simulink model "ECS787"  (R2013a)
settings: Solver=ode45  StartTime=0.0  StopTime=10000  RelTol=1e-3
InitFcn:
  | load('SampleOutput.mat')
  | 
  | load('SampleFuelBurn.mat')
undefined symbols (not defined in the file): AirProp
libraries: PowerFlowLib x8, simulink x4
(part 1 of 6)
settings Model: Creator=ASELab1  LastModifiedBy=ASELab1
settings DataIOCC: SignalLoggingSaveFormat=ModelDataLogs
settings DebuggingCC: MultiTaskDSMMsg=warning  MultiTaskCondExecSysMsg=none  StrictBusMsg=None
settings RTWCC: IncludeERTFirstTime=on

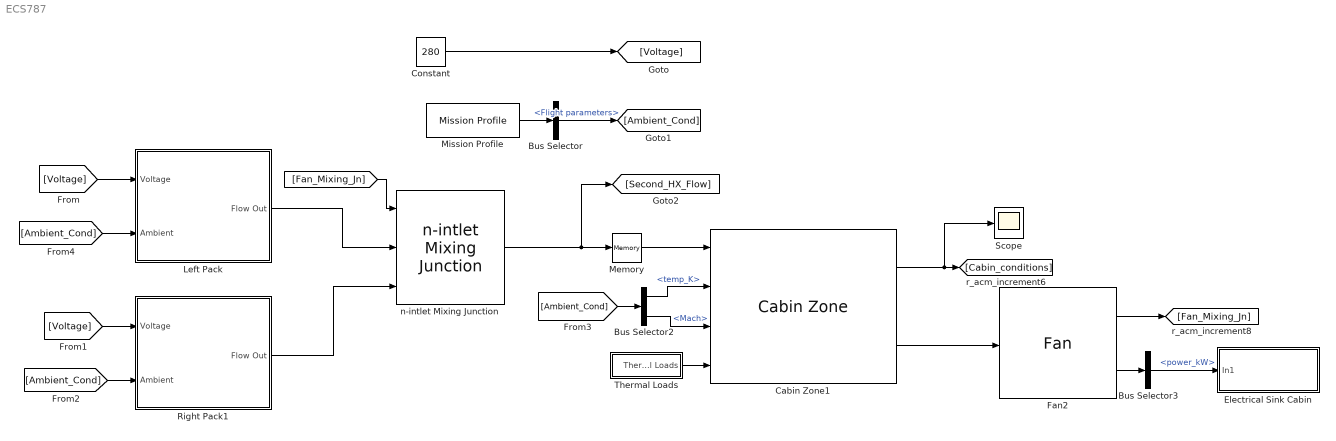
== system ECS787 ==
  Bus Selector : BusSelector  OutputSignals=Flight parameters
  Bus Selector2 : BusSelector  OutputSignals=temp_K,Mach
  Bus Selector3 : BusSelector  OutputSignals=power_kW
  Cabin Zone1 : PowerFlowLib/Energy & Power Systems/Thermal/ECS/Cabin Zone  A_fuselage=880  V_cab=245  n_pass=300  L_shell=0.003  K_shell=1  L_insulation=0.02  K_insulation=1  L_coating=0.002  K_coating=1  Vdot_sa_pass=0.009438  q_pass=60  RAR=.25  h_outside=1  h_inside=1
  Constant : Constant  Value=280
  Electrical Sink Cabin : Subsystem
  Fan2 : PowerFlowLib/Energy & Power Systems/Thermal/ECS/Fan  N_fan=1725
  Left Pack : Subsystem
  Memory : Memory
  Mission Profile : PowerFlowLib/Mission Profile/Mission Profile  mssn_check=off  mssn_prof=MSSN  del_P=0  del_T=0  del_rho=0  pres_msl=101.3  temp_msl=15  dens_msl=1.229
  Right Pack1 : Subsystem
  Scope : Scope
  Thermal Loads : Subsystem
  n-intlet Mixing Junction : PowerFlowLib/Energy & Power Systems/Thermal/ECS/n-intlet Mixing Junction  no_inlets=3  d_in_1=0.1  d_in_2=0.1  d_out=0.2
  wires:
  Mission Profile/1 -> Bus Selector/1
  Constant/1 -> [Voltage]
  Bus Selector/1 -> [Ambient_Cond]  "<Flight parameters>"
  Left Pack/1(Flow Out) -> n-intlet Mixing Junction/2
  Right Pack1/1(Flow Out) -> n-intlet Mixing Junction/3
  n-intlet Mixing Junction/1 -> [Second_HX_Flow], Memory/1
  Memory/1 -> Cabin Zone1/1
  [Ambient_Cond] -> Bus Selector2/1
  Bus Selector2/1 -> Cabin Zone1/2  "<temp_K>"
  Bus Selector2/2 -> Cabin Zone1/3  "<Mach>"
  Thermal Loads/1("Thermal Loads ") -> Cabin Zone1/4
  Cabin Zone1/2 -> Fan2/1
  Cabin Zone1/1 -> Scope/1, [Cabin_conditions]
  Fan2/2 -> Bus Selector3/1
  Bus Selector3/1 -> Electrical Sink Cabin/1(In1)  "<power_kW>"
  Fan2/1 -> [Fan_Mixing_Jn]
  [Fan_Mixing_Jn] -> n-intlet Mixing Junction/1
  [Voltage] -> Left Pack/1(Voltage)
  [Voltage] -> Right Pack1/1(Voltage)
  [Ambient_Cond] -> Left Pack/2(Ambient)
  [Ambient_Cond] -> Right Pack1/2(Ambient)

== system ECS787/Electrical Sink Cabin ==
  In1 : Inport

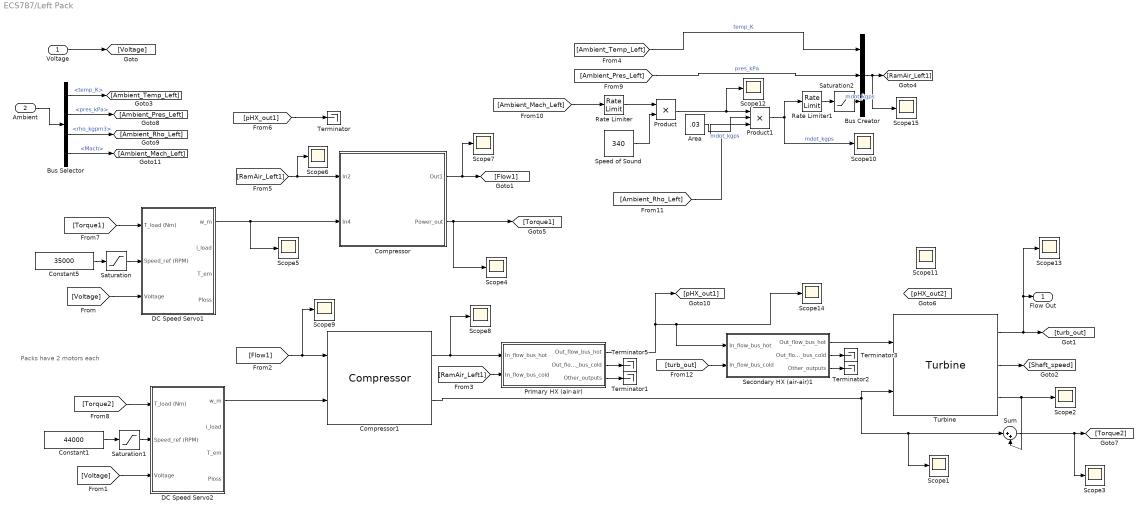
== system ECS787/Left Pack ==
  note: Packs have 2 motors each
  Voltage : Inport
  Ambient : Inport  Port=2
  "Area " : Constant  Value=.03
  Bus Creator : BusCreator  Inputs=3
  Bus Selector : BusSelector  OutputSignals=temp_K,pres_kPa,rho_kgpm3,Mach
  Compressor : Subsystem  AncestorBlock=PowerFlowLib/Energy & Power Systems/Thermal/ECS/Compressor
      mask help: COMPRESSOR (ECS)
      mask init:
      | load AirProp
      | load CompProp
      mask Help:
      | Main Assumptions
      | 1. The Turbine and the compressor are coupled to each other (turbocharger).
      | 2. Maps are provided to compute the efficiency of the compressor.
      | 3. There is no heat transfer from the compressor to the surrounding.
      mask Display:
      | image(imread('compressor.png'))
      | port_label('input',1,'{ \bfFlow In}','texmode','on')
      | port_label('input',2,'{ \bfShaft Speed}','texmode','on');
      | 
      | 
      | port_label('output',1,'{\bfFlow Out}','texmode','on')
      | port_label('output',2,'{\bfComp. Work}','texmode','on')
  Compressor1 : PowerFlowLib/Energy & Power Systems/Thermal/ECS/Compressor
      link override "m and P ": Gain=1
  Constant1 : Constant  Value=44000
  Constant5 : Constant  Value=35000
  DC Speed Servo1 : Subsystem  AncestorBlock=PowerFlowLib/Energy & Power Systems/Electrical/Machines/DC Speed Servo  mask{Vf=280, Ra=0.05, La=0.9e-3, Rfsh=400, Lfsh=320, Lmsh=1.9, J=1.5}
      mask prompts: Vf "Field voltage (V)"; Ra "Armature resistance (Ohms)"; La "Armature inductance (H)"; Rfsh "Shunt field resistance (Ohms)"; Lfsh "Shunt field inductance (H)"; Lmsh "Mutual inductance (H)"; J "Rotor moment of inertia (Kgm^2)"
  DC Speed Servo2 : Subsystem  AncestorBlock=PowerFlowLib/Energy & Power Systems/Electrical/Machines/DC Speed Servo  mask{Vf=280, Ra=0.05, La=0.9e-3, Rfsh=400, Lfsh=320, Lmsh=1.9, J=1.5}
      mask prompts: Vf "Field voltage (V)"; Ra "Armature resistance (Ohms)"; La "Armature inductance (H)"; Rfsh "Shunt field resistance (Ohms)"; Lfsh "Shunt field inductance (H)"; Lmsh "Mutual inductance (H)"; J "Rotor moment of inertia (Kgm^2)"
  Primary HX (air-air) : Subsystem  AncestorBlock=PowerFlowLib/Energy & Power Systems/Thermal/ECS/Air-Air HX  mask(Air-Air Heat Exchanger){L_hx=0.2, W_hx=0.2, H_hx=0.2, t_p=0.0008, K_p=167, cp_hx=883, m_cm=16, l_fin=.005, t_fin=0.0002, s_fin=0.0015, h_fin=0.0095, K_n=167, eta_f=0.8, T_cm_0=50}
      mask prompts: L_hx "Length of HX in the flow direction [m]"; W_hx "Width of HX [m]"; H_hx "Height of HX [m]"; t_p "HX plate thickness [m]"; K_p "Thermal conductivity of the plates [W/m.K]"; cp_hx "Specific heat of the HX material [J/kg.K]"; m_cm "Mass of HX [kg]"; l_fin "Fin length [m]"; t_fin "Fin thickness [m]"; s_fin "Fin free flow width [m]"; h_fin "Fin free flow height [m]"; K_n "Thermal conductivity of the fin material [W/m.K]"; eta_f "Fin efficiency"; T_cm_0 "Initial_HX_core_temp_[C]"
      mask init:
      | load AirProp
      mask Help:
      | Main Assumptions:
      | 
      | 1. Rectangular offset-strip fin heat exchanger.
      | 2. Lumped parameter model.
      | 3. Constant user-defined efficiency.
      | 4. Number of passages is the same for both the cold and hot fluid passages (usually
      | one of the flows has 1 more passage to reduce ambient losses).
      | 5. Similar plate and fin geometries for both the hot and cold fluid sides (the
      | objective is to simplify modeling and reduce the number of input parameters needed).
      | 6. Neglect heat transfer from fin face
      | 7. Neglect conduction heat transfer in the fin and plate bases
      mask Display:
      | port_label('input',1,'{ \bfFlow In (Hot)}','texmode','on')
      | port_label('input',2,'{ \bfFlow In (Cold)}','texmode','on');
      | 
      | port_label('output',1,'{\bfFlow Out (Hot)}','texmode','on')
      | port_label('output',2,'{\bfFlow Out (Cold)}','texmode','on')
      | port_label('output',3,'{\bfMisc. Data}','texmode','on')
  Product : Product
  Product1 : Product  Inputs=3
  Rate Limiter : RateLimiter  RisingSlewLimit=.02  FallingSlewLimit=-.02  SampleTimeMode=inherited
  Rate Limiter1 : RateLimiter  RisingSlewLimit=.02  FallingSlewLimit=-.02  SampleTimeMode=inherited
  Saturation : Saturate  UpperLimit=40000  LowerLimit=10000
  Saturation1 : Saturate  UpperLimit=60000  LowerLimit=30000
  Saturation2 : Saturate  UpperLimit=20  LowerLimit=.01
  Scope{1..15} (15 alike) : Scope
      Scope1 settings: YMin=469600  YMax=470800  SaveName=ScopeData6
      Scope10 settings: YMin=0  YMax=0.25  SaveName=ScopeData17
      Scope11 settings: YMin=-1750  YMax=500
      Scope12 settings: SaveName=ScopeData19
      Scope13 settings: YMin=0  YMax=750  SaveName=ScopeData2
      Scope14 settings: YMin=0  YMax=375  SaveName=ScopeData4
      Scope15 settings: YMin=0  YMax=300  SaveName=ScopeData5
      Scope2 settings: YMin=-2.5e+06  YMax=4e+06  SaveName=ScopeData7
      Scope3 settings: YMin=4.29e+06  YMax=4.3e+06  SaveName=ScopeData8
      Scope4 settings: SaveName=ScopeData9
      Scope5 settings: YMin=0  YMax=11000  SaveName=ScopeData10
      Scope6 settings: SaveName=ScopeData11
      Scope7 settings: TimeRange=10000  YMin=0  YMax=350  SaveName=ScopeData12
      Scope8 settings: YMin=0  YMax=850  SaveName=ScopeData13
      Scope9 settings: YMin=0  YMax=350  SaveName=ScopeData14
  Secondary HX (air-air)1 : Subsystem  AncestorBlock=PowerFlowLib/Energy & Power Systems/Thermal/ECS/Air-Air HX  mask(Air-Air Heat Exchanger){L_hx=0.2, W_hx=0.2, H_hx=0.2, t_p=0.0008, K_p=167, cp_hx=883, m_cm=16, l_fin=.005, t_fin=0.0002, s_fin=0.0015, h_fin=0.0095, K_n=167, eta_f=0.8, T_cm_0=50}
      mask prompts: L_hx "Length of HX in the flow direction [m]"; W_hx "Width of HX [m]"; H_hx "Height of HX [m]"; t_p "HX plate thickness [m]"; K_p "Thermal conductivity of the plates [W/m.K]"; cp_hx "Specific heat of the HX material [J/kg.K]"; m_cm "Mass of HX [kg]"; l_fin "Fin length [m]"; t_fin "Fin thickness [m]"; s_fin "Fin free flow width [m]"; h_fin "Fin free flow height [m]"; K_n "Thermal conductivity of the fin material [W/m.K]"; eta_f "Fin efficiency"; T_cm_0 "Initial_HX_core_temp_[C]"
      mask init:
      | load AirProp
      mask Help:
      | Main Assumptions:
      | 
      | 1. Rectangular offset-strip fin heat exchanger.
      | 2. Lumped parameter model.
      | 3. Constant user-defined efficiency.
      | 4. Number of passages is the same for both the cold and hot fluid passages (usually
      | one of the flows has 1 more passage to reduce ambient losses).
      | 5. Similar plate and fin geometries for both the hot and cold fluid sides (the
      | objective is to simplify modeling and reduce the number of input parameters needed).
      | 6. Neglect heat transfer from fin face
      | 7. Neglect conduction heat transfer in the fin and plate bases
      mask Display:
      | port_label('input',1,'{ \bfFlow In (Hot)}','texmode','on')
      | port_label('input',2,'{ \bfFlow In (Cold)}','texmode','on');
      | 
      | port_label('output',1,'{\bfFlow Out (Hot)}','texmode','on')
      | port_label('output',2,'{\bfFlow Out (Cold)}','texmode','on')
      | port_label('output',3,'{\bfMisc. Data}','texmode','on')
  Speed of Sound : Constant  Value=340
  Sum : Sum  Inputs=|++
  Terminator{,1..3,5} (5 alike) : Terminator
  Turbine : PowerFlowLib/Energy & Power Systems/Thermal/ECS/Turbine  press_Turbine_exit=80  inertia=5e-5  n_t=0.7
  Flow Out : Outport
  wires:
  [Voltage] -> DC Speed Servo1/3(Voltage)
  Constant5/1 -> Saturation/1
  DC Speed Servo1/1(w_m) -> Scope5/1, Compressor/2(In4)
  Compressor/1(Out1) -> Scope7/1, [Flow1]
  [RamAir_Left1] -> Scope6/1, Compressor/1(In2)
  Voltage/1 -> [Voltage]
  [Voltage] -> DC Speed Servo2/3(Voltage)
  Constant1/1 -> Saturation1/1
  DC Speed Servo2/1(w_m) -> Compressor1/2
  [Flow1] -> Scope9/1, Compressor1/1
  [RamAir_Left1] -> Primary HX (air-air)/2(In_flow_bus_cold)
  Compressor1/1 -> Scope8/1, Primary HX (air-air)/1(In_flow_bus_hot)
  ? -> [pHX_out2], Scope11/1
  Primary HX (air-air)/2(Out_flow_bus_cold) -> Terminator5/1
  Primary HX (air-air)/3(Other_outputs) -> Terminator1/1
  Primary HX (air-air)/1(Out_flow_bus_hot) -> Scope14/1, Secondary HX (air-air)1/1(In_flow_bus_hot), [pHX_out1]
  Turbine/2 -> [Shaft_speed]
  Turbine/1 -> Scope13/1, Flow Out/1, [turb_out]
  Ambient/1 -> Bus Selector/1
  [pHX_out1] -> Terminator/1
  Bus Creator/1 -> Scope15/1, [RamAir_Left1]
  Bus Selector/1 -> [Ambient_Temp_Left]  "<temp_K>"
  Saturation/1 -> DC Speed Servo1/2(Speed_ref (RPM))
  Saturation1/1 -> DC Speed Servo2/2(Speed_ref (RPM))
  Compressor/2(Power_out) -> [Torque1], Scope4/1
  [Torque1] -> DC Speed Servo1/1(T_load (Nm))
  Compressor1/2 -> Turbine/2, Scope1/1, Sum/1
  Sum/1 -> Scope3/1, [Torque2]
  [Torque2] -> DC Speed Servo2/1(T_load (Nm))
  Turbine/3 -> Sum/2, Scope2/1
  [Ambient_Temp_Left] -> Bus Creator/1  "temp_K"
  [Ambient_Pres_Left] -> Bus Creator/2  "pres_kPa"
  Product1/1 -> Rate Limiter1/1, Scope10/1  "mdot_kgps"
  Bus Selector/2 -> [Ambient_Pres_Left]  "<pres_kPa>"
  Bus Selector/3 -> [Ambient_Rho_Left]  "<rho_kgpm3>"
  Bus Selector/4 -> [Ambient_Mach_Left]  "<Mach>"
  Speed of Sound/1 -> Product/2
  [Ambient_Rho_Left] -> Product1/3
  Product/1 -> Product1/1, Scope12/1
  [Ambient_Mach_Left] -> Rate Limiter/1
  "Area "/1 -> Product1/2  "mdot_kgps"
  Saturation2/1 -> Bus Creator/3  "mdot_kgps"
  [turb_out] -> Secondary HX (air-air)1/2(In_flow_bus_cold)
  Secondary HX (air-air)1/1(Out_flow_bus_hot) -> Turbine/1
  Secondary HX (air-air)1/2(Out_flow_bus_cold) -> Terminator3/1
  Secondary HX (air-air)1/3(Other_outputs) -> Terminator2/1
  Rate Limiter/1 -> Product/1
  Rate Limiter1/1 -> Saturation2/1

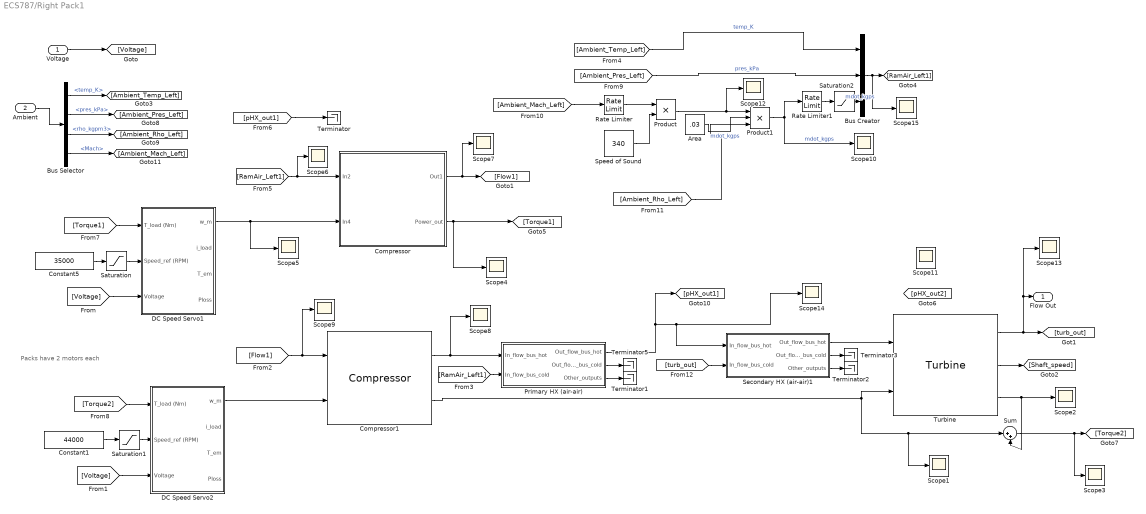
== system ECS787/Right Pack1 ==
  note: Packs have 2 motors each
  Voltage : Inport
  Ambient : Inport  Port=2
  "Area " : Constant  Value=.03
  Bus Creator : BusCreator  Inputs=3
  Bus Selector : BusSelector  OutputSignals=temp_K,pres_kPa,rho_kgpm3,Mach
  Compressor : Subsystem  AncestorBlock=PowerFlowLib/Energy & Power Systems/Thermal/ECS/Compressor
      mask help: COMPRESSOR (ECS)
      mask init:
      | load AirProp
      | load CompProp
      mask Help:
      | Main Assumptions
      | 1. The Turbine and the compressor are coupled to each other (turbocharger).
      | 2. Maps are provided to compute the efficiency of the compressor.
      | 3. There is no heat transfer from the compressor to the surrounding.
      mask Display:
      | image(imread('compressor.png'))
      | port_label('input',1,'{ \bfFlow In}','texmode','on')
      | port_label('input',2,'{ \bfShaft Speed}','texmode','on');
      | 
      | 
      | port_label('output',1,'{\bfFlow Out}','texmode','on')
      | port_label('output',2,'{\bfComp. Work}','texmode','on')
  Compressor1 : PowerFlowLib/Energy & Power Systems/Thermal/ECS/Compressor
      link override "m and P ": Gain=1
  Constant1 : Constant  Value=44000
  Constant5 : Constant  Value=35000
  DC Speed Servo1 : Subsystem  AncestorBlock=PowerFlowLib/Energy & Power Systems/Electrical/Machines/DC Speed Servo  mask{Vf=280, Ra=0.05, La=0.9e-3, Rfsh=400, Lfsh=320, Lmsh=1.9, J=1.5}
      mask prompts: Vf "Field voltage (V)"; Ra "Armature resistance (Ohms)"; La "Armature inductance (H)"; Rfsh "Shunt field resistance (Ohms)"; Lfsh "Shunt field inductance (H)"; Lmsh "Mutual inductance (H)"; J "Rotor moment of inertia (Kgm^2)"
  DC Speed Servo2 : Subsystem  AncestorBlock=PowerFlowLib/Energy & Power Systems/Electrical/Machines/DC Speed Servo  mask{Vf=280, Ra=0.05, La=0.9e-3, Rfsh=400, Lfsh=320, Lmsh=1.9, J=1.5}
      mask prompts: Vf "Field voltage (V)"; Ra "Armature resistance (Ohms)"; La "Armature inductance (H)"; Rfsh "Shunt field resistance (Ohms)"; Lfsh "Shunt field inductance (H)"; Lmsh "Mutual inductance (H)"; J "Rotor moment of inertia (Kgm^2)"
  Primary HX (air-air) : Subsystem  AncestorBlock=PowerFlowLib/Energy & Power Systems/Thermal/ECS/Air-Air HX  mask(Air-Air Heat Exchanger){L_hx=0.2, W_hx=0.2, H_hx=0.2, t_p=0.0008, K_p=167, cp_hx=883, m_cm=16, l_fin=.005, t_fin=0.0002, s_fin=0.0015, h_fin=0.0095, K_n=167, eta_f=0.8, T_cm_0=50}
      mask prompts: L_hx "Length of HX in the flow direction [m]"; W_hx "Width of HX [m]"; H_hx "Height of HX [m]"; t_p "HX plate thickness [m]"; K_p "Thermal conductivity of the plates [W/m.K]"; cp_hx "Specific heat of the HX material [J/kg.K]"; m_cm "Mass of HX [kg]"; l_fin "Fin length [m]"; t_fin "Fin thickness [m]"; s_fin "Fin free flow width [m]"; h_fin "Fin free flow height [m]"; K_n "Thermal conductivity of the fin material [W/m.K]"; eta_f "Fin efficiency"; T_cm_0 "Initial_HX_core_temp_[C]"
      mask init:
      | load AirProp
      mask Help:
      | Main Assumptions:
      | 
      | 1. Rectangular offset-strip fin heat exchanger.
      | 2. Lumped parameter model.
      | 3. Constant user-defined efficiency.
      | 4. Number of passages is the same for both the cold and hot fluid passages (usually
      | one of the flows has 1 more passage to reduce ambient losses).
      | 5. Similar plate and fin geometries for both the hot and cold fluid sides (the
      | objective is to simplify modeling and reduce the number of input parameters needed).
      | 6. Neglect heat transfer from fin face
      | 7. Neglect conduction heat transfer in the fin and plate bases
      mask Display:
      | port_label('input',1,'{ \bfFlow In (Hot)}','texmode','on')
      | port_label('input',2,'{ \bfFlow In (Cold)}','texmode','on');
      | 
      | port_label('output',1,'{\bfFlow Out (Hot)}','texmode','on')
      | port_label('output',2,'{\bfFlow Out (Cold)}','texmode','on')
      | port_label('output',3,'{\bfMisc. Data}','texmode','on')
  Product : Product
  Product1 : Product  Inputs=3
  Rate Limiter : RateLimiter  RisingSlewLimit=.02  FallingSlewLimit=-.02  SampleTimeMode=inherited
  Rate Limiter1 : RateLimiter  RisingSlewLimit=.02  FallingSlewLimit=-.02  SampleTimeMode=inherited
  Saturation : Saturate  UpperLimit=40000  LowerLimit=10000
  Saturation1 : Saturate  UpperLimit=60000  LowerLimit=30000
  Saturation2 : Saturate  UpperLimit=20  LowerLimit=.01
  Scope{1..15} (15 alike) : Scope
      Scope1 settings: YMin=469600  YMax=470800  SaveName=ScopeData6
      Scope10 settings: YMin=0  YMax=0.25  SaveName=ScopeData17
      Scope11 settings: YMin=-1750  YMax=500
      Scope12 settings: SaveName=ScopeData19
      Scope13 settings: YMin=0  YMax=750  SaveName=ScopeData2
      Scope14 settings: YMin=0  YMax=375  SaveName=ScopeData4
      Scope15 settings: YMin=0  YMax=300  SaveName=ScopeData5
      Scope2 settings: YMin=-2.5e+06  YMax=4e+06  SaveName=ScopeData7
      Scope3 settings: YMin=4.29e+06  YMax=4.3e+06  SaveName=ScopeData8
      Scope4 settings: SaveName=ScopeData9
      Scope5 settings: YMin=0  YMax=11000  SaveName=ScopeData10
      Scope6 settings: SaveName=ScopeData11
      Scope7 settings: TimeRange=10000  YMin=0  YMax=350  SaveName=ScopeData12
      Scope8 settings: YMin=0  YMax=850  SaveName=ScopeData13
      Scope9 settings: YMin=0  YMax=350  SaveName=ScopeData14
  Secondary HX (air-air)1 : Subsystem  AncestorBlock=PowerFlowLib/Energy & Power Systems/Thermal/ECS/Air-Air HX  mask(Air-Air Heat Exchanger){L_hx=0.2, W_hx=0.2, H_hx=0.2, t_p=0.0008, K_p=167, cp_hx=883, m_cm=16, l_fin=.005, t_fin=0.0002, s_fin=0.0015, h_fin=0.0095, K_n=167, eta_f=0.8, T_cm_0=50}
      mask prompts: L_hx "Length of HX in the flow direction [m]"; W_hx "Width of HX [m]"; H_hx "Height of HX [m]"; t_p "HX plate thickness [m]"; K_p "Thermal conductivity of the plates [W/m.K]"; cp_hx "Specific heat of the HX material [J/kg.K]"; m_cm "Mass of HX [kg]"; l_fin "Fin length [m]"; t_fin "Fin thickness [m]"; s_fin "Fin free flow width [m]"; h_fin "Fin free flow height [m]"; K_n "Thermal conductivity of the fin material [W/m.K]"; eta_f "Fin efficiency"; T_cm_0 "Initial_HX_core_temp_[C]"
      mask init:
      | load AirProp
      mask Help:
      | Main Assumptions:
      | 
      | 1. Rectangular offset-strip fin heat exchanger.
      | 2. Lumped parameter model.
      | 3. Constant user-defined efficiency.
      | 4. Number of passages is the same for both the cold and hot fluid passages (usually
      | one of the flows has 1 more passage to reduce ambient losses).
      | 5. Similar plate and fin geometries for both the hot and cold fluid sides (the
      | objective is to simplify modeling and reduce the number of input parameters needed).
      | 6. Neglect heat transfer from fin face
      | 7. Neglect conduction heat transfer in the fin and plate bases
      mask Display:
      | port_label('input',1,'{ \bfFlow In (Hot)}','texmode','on')
      | port_label('input',2,'{ \bfFlow In (Cold)}','texmode','on');
      | 
      | port_label('output',1,'{\bfFlow Out (Hot)}','texmode','on')
      | port_label('output',2,'{\bfFlow Out (Cold)}','texmode','on')
      | port_label('output',3,'{\bfMisc. Data}','texmode','on')
  Speed of Sound : Constant  Value=340
  Sum : Sum  Inputs=|++
  Terminator{,1..3,5} (5 alike) : Terminator
  Turbine : PowerFlowLib/Energy & Power Systems/Thermal/ECS/Turbine  press_Turbine_exit=80  inertia=5e-5  n_t=0.7
  Flow Out : Outport
  wires:
  [Voltage] -> DC Speed Servo1/3(Voltage)
  Constant5/1 -> Saturation/1
  DC Speed Servo1/1(w_m) -> Scope5/1, Compressor/2(In4)
  Compressor/1(Out1) -> Scope7/1, [Flow1]
  [RamAir_Left1] -> Scope6/1, Compressor/1(In2)
  Voltage/1 -> [Voltage]
  [Voltage] -> DC Speed Servo2/3(Voltage)
  Constant1/1 -> Saturation1/1
  DC Speed Servo2/1(w_m) -> Compressor1/2
  [Flow1] -> Scope9/1, Compressor1/1
  [RamAir_Left1] -> Primary HX (air-air)/2(In_flow_bus_cold)
  Compressor1/1 -> Scope8/1, Primary HX (air-air)/1(In_flow_bus_hot)
  ? -> [pHX_out2], Scope11/1
  Primary HX (air-air)/2(Out_flow_bus_cold) -> Terminator5/1
  Primary HX (air-air)/3(Other_outputs) -> Terminator1/1
  Primary HX (air-air)/1(Out_flow_bus_hot) -> Scope14/1, Secondary HX (air-air)1/1(In_flow_bus_hot), [pHX_out1]
  Turbine/2 -> [Shaft_speed]
  Turbine/1 -> Scope13/1, Flow Out/1, [turb_out]
  Ambient/1 -> Bus Selector/1
  [pHX_out1] -> Terminator/1
  Bus Creator/1 -> Scope15/1, [RamAir_Left1]
  Bus Selector/1 -> [Ambient_Temp_Left]  "<temp_K>"
  Saturation/1 -> DC Speed Servo1/2(Speed_ref (RPM))
  Saturation1/1 -> DC Speed Servo2/2(Speed_ref (RPM))
  Compressor/2(Power_out) -> [Torque1], Scope4/1
  [Torque1] -> DC Speed Servo1/1(T_load (Nm))
  Compressor1/2 -> Turbine/2, Scope1/1, Sum/1
  Sum/1 -> Scope3/1, [Torque2]
  [Torque2] -> DC Speed Servo2/1(T_load (Nm))
  Turbine/3 -> Sum/2, Scope2/1
  [Ambient_Temp_Left] -> Bus Creator/1  "temp_K"
  [Ambient_Pres_Left] -> Bus Creator/2  "pres_kPa"
  Product1/1 -> Rate Limiter1/1, Scope10/1  "mdot_kgps"
  Bus Selector/2 -> [Ambient_Pres_Left]  "<pres_kPa>"
  Bus Selector/3 -> [Ambient_Rho_Left]  "<rho_kgpm3>"
  Bus Selector/4 -> [Ambient_Mach_Left]  "<Mach>"
  Speed of Sound/1 -> Product/2
  [Ambient_Rho_Left] -> Product1/3
  Product/1 -> Product1/1, Scope12/1
  [Ambient_Mach_Left] -> Rate Limiter/1
  "Area "/1 -> Product1/2  "mdot_kgps"
  Saturation2/1 -> Bus Creator/3  "mdot_kgps"
  [turb_out] -> Secondary HX (air-air)1/2(In_flow_bus_cold)
  Secondary HX (air-air)1/1(Out_flow_bus_hot) -> Turbine/1
  Secondary HX (air-air)1/2(Out_flow_bus_cold) -> Terminator3/1
  Secondary HX (air-air)1/3(Other_outputs) -> Terminator2/1
  Rate Limiter/1 -> Product/1
  Rate Limiter1/1 -> Saturation2/1

== system ECS787/Thermal Loads ==
  "Thermal Loads " : Outport

== system ECS787/Left Pack/Compressor ==
  note: Flow
  note: N
  note: eff
  In2 : Inport
  In4 : Inport  Port=2
  Add : Sum
  Bias : Bias  Bias=-1
  Bus Creator1 : BusCreator  Inputs=3
  Bus Selector : BusSelector  OutputSignals=pres_kPa
  Bus Selector1 : BusSelector  OutputSignals=mdot_kgps
  Bus Selector2 : BusSelector  OutputSignals=temp_K
  Cp(P,T)1 : Lookup_n-D  BreakpointsForDimension1=AirProp.P  BreakpointsForDimension2=AirProp.T  BreakpointsForDimension3=[1]  Table=AirProp.Cp_pt  RndMeth=Simplest  InputSameDT=on
  Divide1 : Product  Inputs=/**
  Divide2 : Product  Inputs=***
  Divide3 : Product  Inputs=**
  Divide4 : Product  Inputs=/*
  Divide5 : Product  Inputs=/**
  Gain1 : Gain  Gain=1000
  K to R : Gain  Gain=1.8
  Math Function : Math  Operator=pow  SaturateOnIntegerOverflow=on
  Pressure_ratio : Lookup_n-D  BreakpointsForDimension1=[20,25,30,35,40,45,50,55,60,65,70,75,80,85,90]  BreakpointsForDimension2=[1097,1316,1536,1756,1975,2195,2414]  Table=reshape([1.22,1.202,1.18,1.145,1.05,1,1,1,1,1,1,1,1,1,1,1.325,1.31,1.3,1.275,1.22,1.16,1,1,1,1,1,1,1,1,1,1.49,1.485,1.475,1.45,1.41,1.38,1.3,1.15,1,1,1,1,1,1,1,1.65,1.65,1.63,1.628,1.61,1.598,1.55,1.5,1.4,1.1,1,1,1,1,1,1.885,1.87,1.87,1.86,1.83,1.82,1.8,1.76,1.7,1.62,1.5,1,1,1,1,2.15,2.15,2.15,2.14,2.12,2.05,2.085,2.05,2.01,1.98,1.902,1.8,1,1,1,2.45,2.44,2.43,2.42,2.41,2.405,2.4,2.39,2.365,2.32,2.28,2.2,2.14,2.02,1.7],15,7)  RndMeth=Simplest  InputSameDT=on
  Reciprocal Sqrt : Sqrt  SaturateOnIntegerOverflow=on
  Scope1 : Scope
      settings: SaveName=ScopeData16
  Scope5 : Scope
      settings: SaveName=ScopeData15
  Table1 : Lookup_n-D  BreakpointsForDimension1=[20,25,30,35,40,45,50,55,60,65,70,75,80,85,90]  BreakpointsForDimension2=[1097,1316,1536,1756,1975,2195,2414]  Table=reshape([0.84396,0.83224,0.7928,0.70795,0.33,0.16,0.16,0.16,0.16,0.16,0.16,0.16,0.16,0.16,0.16,0.8265,0.8272,0.823,0.8075,0.709,0.5437,0.0850000000000002,0.0850000000000002,0.0850000000000002,0.0850000000000002,0.0850000000000002,0.0850000000000002,0.0850000000000002,0.0850000000000002,0.0850000000000002,0.6962,0.716699999999999,0.753,0.8086,0.8094,0.777,0.672,0.3705,0.0690000000000002,0.0690000000000002,0.0690000000000002,0.0690000000000002,0.0690000000000002,0.0690000000000002,0.0690000000000002,0.803,0.803,0.8122,0.81312,0.82042,0.822052,0.8045,0.755,0.654,0.192,0.0480000000000002,0.0480000000000002,0.0480000000000002,0.0480000000000002,0.0480000000000002,0.79155,0.8025,0.8025,0.806,0.81335,0.8144,0.8165,0.811,0.7775,0.7328,0.628,0.0080000000000004,0.0080000000000004,0.0080000000000004,0.0080000000000004,0.802,0.802,0.802,0.802,0.802,0.8112,0.80584,0.8112,0.81728,0.80648,0.77466,0.723,0.00180000000000019,0.00180000000000019,0.00180000000000019,0.81,0.81,0.81,0.81,0.81,0.81,0.81,0.81,0.81,0.81,0.8068,0.7888,0.766,0.72408,0.54796],15,7)  RndMeth=Simplest  InputSameDT=on
  "m and P " : Gain
  poly index : Constant  Value=(1.4-1)/1.4
  Out1 : Outport
  Power_out : Outport  Port=2
  wires:
  Gain1/1 -> Divide2/2
  Cp(P,T)1/1 -> Gain1/1
  In2/1 -> Bus Selector/1, Bus Selector1/1, Bus Selector2/1
  Bus Selector2/1 -> Divide1/3, Add/2, K to R/1  "<temp_K>"
  Reciprocal Sqrt/1 -> Divide4/1, Divide5/3
  Bus Selector1/1 -> Divide2/1, Bus Creator1/2, Divide5/2  "<mdot_kgps>"
  Pressure_ratio/1 -> Math Function/1, Divide3/2
  poly index/1 -> Math Function/2
  Math Function/1 -> Bias/1
  Bias/1 -> Divide1/2
  Divide1/1 -> Cp(P,T)1/2, Divide2/3, Add/1
  Divide2/1 -> Power_out/1
  Bus Selector/1 -> Divide3/1, Divide5/1  "<pres_kPa>"
  Divide3/1 -> Cp(P,T)1/1, Bus Creator1/1  "pres_kPa"
  Add/1 -> Bus Creator1/3  "temp_K"
  Bus Creator1/1 -> Out1/1
  K to R/1 -> Reciprocal Sqrt/1
  In4/1 -> Scope1/1, Divide4/2
  Divide4/1 -> Scope5/1, Pressure_ratio/2, Table1/2
  Divide5/1 -> "m and P "/1
  "m and P "/1 -> Pressure_ratio/1, Table1/1
  Table1/1 -> Divide1/1

== system ECS787/Left Pack/DC Speed Servo1 ==
  T_load (Nm) : Inport
  Speed_ref (RPM) : Inport  Port=2
  Voltage : Inport  Port=3
  DC Machine : Subsystem
  Fcn : Fcn  Expr=u(1)/(u(2)+0.1)
  Gain2 : Gain  Gain=60/(2*pi)
  Mux : Mux  Inputs=2
  PID Controller : simulink/Continuous/PID Controller  Controller=PID  TimeDomain=Continuous-time  SampleTime=1  IntegratorMethod=Forward Euler  FilterMethod=Forward Euler  Form=Parallel  P=1  I=0.1  D=0  N=100  InitialConditionSource=internal  InitialConditionForIntegrator=0  InitialConditionForFilter=0  ExternalReset=none  LimitOutput=off  UpperSaturationLimit=inf  LowerSaturationLimit=-inf  LinearizeAsGain=on  AntiWindupMode=none  Kb=1  TrackingMode=off  Kt=1  PParamMin=[]  PParamMax=[]  IParamMin=[]  IParamMax=[]  DParamMin=[]  DParamMax=[]  NParamMin=[]  NParamMax=[]  KbParamMin=[]  KbParamMax=[]  KtParamMin=[]  KtParamMax=[]  POutMin=[]  POutMax=[]  IOutMin=[]  IOutMax=[]  DOutMin=[]  DOutMax=[]  NOutMin=[]  NOutMax=[]  KbOutMin=[]  KbOutMax=[]  KtOutMin=[]  KtOutMax=[]  IntegratorOutMin=[]  IntegratorOutMax=[]  FilterOutMin=[]  FilterOutMax=[]  SumOutMin=[]  SumOutMax=[]  SumI1OutMin=[]  SumI1OutMax=[]  SumI2OutMin=[]  SumI2OutMax=[]  SumI3OutMin=[]  SumI3OutMax=[]  SumDOutMin=[]  SumDOutMax=[]  SaturationOutMin=[]  SaturationOutMax=[]  IntegratorContinuousStateAttributes=''  IntegratorStateMustResolveToSignalObject=off  IntegratorRTWStateStorageClass=Auto  FilterContinuousStateAttributes=''  FilterStateMustResolveToSignalObject=off  FilterRTWStateStorageClass=Auto
  Sum : Sum  Inputs=-+|
  Terminator{,1..3} (4 alike) : Terminator
  w_m : Outport
  i_load : Outport  Port=2
  T_em : Outport  Port=3
  Ploss : Outport  Port=4
  wires:
  DC Machine/5(Plosses) -> Ploss/1
  Sum/1 -> PID Controller/1
  Gain2/1 -> Sum/1, w_m/1
  Speed_ref (RPM)/1 -> Sum/2
  T_load (Nm)/1 -> DC Machine/3(Tload)
  DC Machine/6(Te) -> T_em/1
  Mux/1 -> Fcn/1
  DC Machine/3(Pe) -> Mux/1
  Fcn/1 -> i_load/1
  DC Machine/7(Speed) -> Gain2/1
  Voltage/1 -> DC Machine/1(Vf), Mux/2
  PID Controller/1 -> DC Machine/2(Va)
  DC Machine/1(If) -> Terminator/1
  DC Machine/2(Ia) -> Terminator1/1
  DC Machine/4(Pm) -> Terminator2/1
  DC Machine/8(theta) -> Terminator3/1

== system ECS787/Left Pack/DC Speed Servo2 ==
  T_load (Nm) : Inport
  Speed_ref (RPM) : Inport  Port=2
  Voltage : Inport  Port=3
  DC Machine : Subsystem
  Fcn : Fcn  Expr=u(1)/(u(2)+0.1)
  Gain2 : Gain  Gain=60/(2*pi)
  Mux : Mux  Inputs=2
  PID Controller : simulink/Continuous/PID Controller  Controller=PID  TimeDomain=Continuous-time  SampleTime=1  IntegratorMethod=Forward Euler  FilterMethod=Forward Euler  Form=Parallel  P=1  I=0.1  D=0  N=100  InitialConditionSource=internal  InitialConditionForIntegrator=0  InitialConditionForFilter=0  ExternalReset=none  LimitOutput=off  UpperSaturationLimit=inf  LowerSaturationLimit=-inf  LinearizeAsGain=on  AntiWindupMode=none  Kb=1  TrackingMode=off  Kt=1  PParamMin=[]  PParamMax=[]  IParamMin=[]  IParamMax=[]  DParamMin=[]  DParamMax=[]  NParamMin=[]  NParamMax=[]  KbParamMin=[]  KbParamMax=[]  KtParamMin=[]  KtParamMax=[]  POutMin=[]  POutMax=[]  IOutMin=[]  IOutMax=[]  DOutMin=[]  DOutMax=[]  NOutMin=[]  NOutMax=[]  KbOutMin=[]  KbOutMax=[]  KtOutMin=[]  KtOutMax=[]  IntegratorOutMin=[]  IntegratorOutMax=[]  FilterOutMin=[]  FilterOutMax=[]  SumOutMin=[]  SumOutMax=[]  SumI1OutMin=[]  SumI1OutMax=[]  SumI2OutMin=[]  SumI2OutMax=[]  SumI3OutMin=[]  SumI3OutMax=[]  SumDOutMin=[]  SumDOutMax=[]  SaturationOutMin=[]  SaturationOutMax=[]  IntegratorContinuousStateAttributes=''  IntegratorStateMustResolveToSignalObject=off  IntegratorRTWStateStorageClass=Auto  FilterContinuousStateAttributes=''  FilterStateMustResolveToSignalObject=off  FilterRTWStateStorageClass=Auto
  Sum : Sum  Inputs=-+|
  Terminator{,1..3} (4 alike) : Terminator
  w_m : Outport
  i_load : Outport  Port=2
  T_em : Outport  Port=3
  Ploss : Outport  Port=4
  wires:
  DC Machine/5(Plosses) -> Ploss/1
  Sum/1 -> PID Controller/1
  Gain2/1 -> Sum/1, w_m/1
  Speed_ref (RPM)/1 -> Sum/2
  T_load (Nm)/1 -> DC Machine/3(Tload)
  DC Machine/6(Te) -> T_em/1
  Mux/1 -> Fcn/1
  DC Machine/3(Pe) -> Mux/1
  Fcn/1 -> i_load/1
  DC Machine/7(Speed) -> Gain2/1
  Voltage/1 -> DC Machine/1(Vf), Mux/2
  PID Controller/1 -> DC Machine/2(Va)
  DC Machine/1(If) -> Terminator/1
  DC Machine/2(Ia) -> Terminator1/1
  DC Machine/4(Pm) -> Terminator2/1
  DC Machine/8(theta) -> Terminator3/1

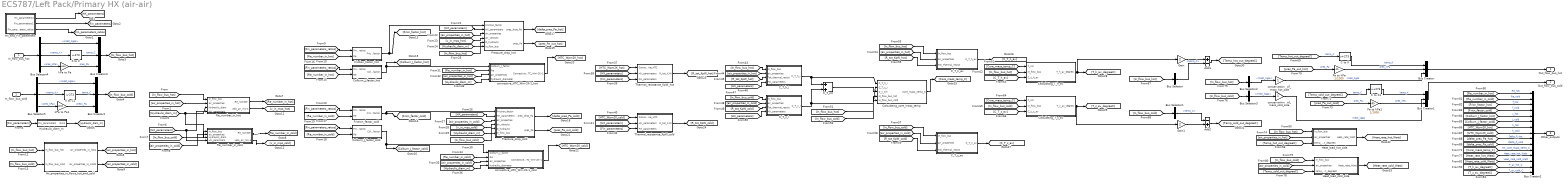
== system ECS787/Left Pack/Primary HX (air-air) ==
  In_flow_bus_hot : Inport
  In_flow_bus_cold : Inport  Port=2
  Add1 : Sum  Inputs=+-
  Add2 : Sum  Inputs=-+
  Air_properties_in_flows_hot_and_cold : Subsystem
  Bus Creator{,1,3..4} (4 alike) : BusCreator  Inputs=3
  Bus Creator2 : BusCreator  Inputs=15
  Bus Selector : BusSelector  OutputSignals=temp_C
  Bus Selector1 : BusSelector  OutputSignals=temp_C
  Bus Selector2 : BusSelector  OutputSignals=mdot_kgps
  Bus Selector3 : BusSelector  OutputSignals=mdot_kgps
  Bus Selector4 : BusSelector  OutputSignals=mdot_kgps,temp_K,pres_kPa
  Bus Selector5 : BusSelector  OutputSignals=mdot_kgps,temp_K,pres_kPa
  C to K : Bias  Bias=273
  C to K1 : Bias  Bias=273
  C_T_c_av : Subsystem
  C_T_c_i : Subsystem
  C_T_cm : Sum
  C_T_h_av : Subsystem
  C_T_h_i : Subsystem
  Calculating_T_c_av : Subsystem
  Calculating_T_h_av : Subsystem
  Calculating_core_mass_temp : Subsystem
  Colburn_J_factor_cold : Subsystem
  Colburn_J_factor_hot : Subsystem
  Friction_factor_cold : Subsystem
  Friction_factor_hot : Subsystem
  Gain : Gain  Gain=2
  Gain1 : Gain  Gain=2
  HX_and_Fin_paramters : Subsystem
  Heat_load_cold_side : Subsystem
  Heat_load_hot_side : Subsystem
  Hydraulic_diam_m : Subsystem
  K to C : Bias  Bias=-273
  K to C1 : Bias  Bias=-273
  Pa to kPa : Gain  Gain=1/1000
  Pa to kPa1 : Gain  Gain=1/1000
  Pressure_drop_cold : Subsystem
  Pressure_drop_hot : Subsystem
  Re_number_in_cold : Subsystem
  Re_number_in_hot : Subsystem
  Thermal_resistance_KpW_cold : Subsystem
  Thermal_resistance_KpW_hot : Subsystem
  conservation _of_mass_cold_side : Gain
  conservation _of_mass_hot_side : Gain
  convective_HTC_Wm-2K-1_cold : Subsystem
  convective_HTC_Wm-2K-1_hot : Subsystem
  kPa to Pa : Gain  Gain=1000
  kPa to Pa1 : Gain  Gain=1000
  Out_flow_bus_hot : Outport
  Out_flow_bus_cold : Outport  Port=2
  Other_outputs : Outport  Port=3
  wires:
  Heat_load_cold_side/1(Heat_rate_Watt) -> [Heat_rate_cold_Watt]
  [air_properties_in_cold] -> Heat_load_cold_side/2(air_properties)
  [In_flow_bus_cold] -> Heat_load_cold_side/1(In_flow_bus)
  [Temp_cold_out_degreeC] -> Heat_load_cold_side/3(temp_out_degreeC)
  Heat_load_hot_side/1(Heat_rate_Watt) -> [Heat_rate_hot_Watt]
  [air_properties_in_hot] -> Heat_load_hot_side/2(air_properties)
  [In_flow_bus_hot] -> Heat_load_hot_side/1(In_flow_bus)
  [Temp_hot_out_degreeC] -> Heat_load_hot_side/3(temp_out_degreeC)
  [R_tot_KpW_cold] -> C_T_c_av/3(Tot_thermal_resist)
  [air_properties_in_cold] -> C_T_c_av/2(air_properties)
  [In_flow_bus_cold] -> C_T_c_av/1(In_flow_bus)
  C_T_c_av/1(C_T_c_av) -> [C_T_c_av]
  Re_number_in_cold/2(velo_air_ms-1) -> [v_in_mps_cold]
  Bus Creator2/1 -> Other_outputs/1
  Bus Creator1/1 -> Out_flow_bus_cold/1
  Bus Creator/1 -> Out_flow_bus_hot/1
  conservation _of_mass_cold_side/1 -> Bus Creator1/3  "mdot_kgps"
  Bus Selector3/1 -> conservation _of_mass_cold_side/1  "<mdot_kgps>"
  conservation _of_mass_hot_side/1 -> Bus Creator/3  "mdot_kgps"
  Bus Selector2/1 -> conservation _of_mass_hot_side/1  "<mdot_kgps>"
  [In_flow_bus_cold] -> Bus Selector3/1
  [In_flow_bus_hot] -> Bus Selector2/1
  [pres_Pa_out_cold] -> Pa to kPa1/1  "pres_Pa"
  [Temp_cold_out_degreeC] -> C to K1/1  "temp_C"
  [pres_Pa_out_hot] -> Pa to kPa/1  "pres_Pa"
  [Temp_hot_out_degreeC] -> C to K/1  "temp_C"
  Add2/1 -> [Temp_cold_out_degreeC]
  Add1/1 -> [Temp_hot_out_degreeC]
  Bus Selector1/1 -> Add2/1  "<temp_C>"
  Gain1/1 -> Add2/2
  Bus Selector/1 -> Add1/2  "<temp_C>"
  Gain/1 -> Add1/1
  [In_flow_bus_cold] -> Bus Selector1/1
  [In_flow_bus_hot] -> Bus Selector/1
  Calculating_T_h_av/1(T_h_av_degreC) -> Gain/1, [T_h_av_degreeC]
  Calculating_T_c_av/1(T_c_av_degreC) -> Gain1/1, [T_c_av_degreeC]
  [C_T_c_av] -> Calculating_T_c_av/3(C_t_c_av)
  [In_flow_bus_cold] -> Calculating_T_c_av/2(In_flow_bus)
  [Core_mass_temp_C] -> Calculating_T_c_av/1(T_cm)
  [C_T_h_av] -> Calculating_T_h_av/3(C_t_h_av)
  C_T_h_av/1(C_T_h_av) -> [C_T_h_av]
  [In_flow_bus_hot] -> Calculating_T_h_av/2(In_flow_bus)
  [Core_mass_temp_C] -> Calculating_T_h_av/1(T_cm)
  Calculating_core_mass_temp/1(Core_mass_temp_C) -> [Core_mass_temp_C]
  [R_tot_KpW_hot] -> C_T_h_av/3(Tot_thermal_resist)
  [air_properties_in_hot] -> C_T_h_av/2(air_properties)
  [In_flow_bus_hot] -> C_T_h_av/1(In_flow_bus)
  [In_flow_bus_cold] -> Calculating_core_mass_temp/5(In_flow_bus_cold)
  [In_flow_bus_hot] -> Calculating_core_mass_temp/4(In_flow_bus_hot)
  C_T_cm/1 -> Calculating_core_mass_temp/3(C_t_cm)
  C_T_c_i/1(C_T_c_i) -> Calculating_core_mass_temp/2(C_T_c_i), C_T_cm/2
  C_T_h_i/1(C_T_h_i) -> Calculating_core_mass_temp/1(C_T_h_i), C_T_cm/1
  [HX_parameters] -> C_T_c_i/4(HX_parameters)
  [R_tot_KpW_cold] -> C_T_c_i/3(Tot_thermal_resist)
  [air_properties_in_cold] -> C_T_c_i/2(air_properties)
  [In_flow_bus_cold] -> C_T_c_i/1(In_flow_bus)
  [HX_parameters] -> C_T_h_i/4(HX_parameters)
  [R_tot_KpW_hot] -> C_T_h_i/3(Tot_thermal_resist)
  Thermal_resistance_KpW_cold/1(R_tot_K/W) -> [R_tot_KpW_cold]
  Thermal_resistance_KpW_hot/1(R_tot_K/W) -> [R_tot_KpW_hot]
  [air_properties_in_hot] -> C_T_h_i/2(air_properties)
  [In_flow_bus_hot] -> C_T_h_i/1(In_flow_bus)
  [HX_parameters] -> Thermal_resistance_KpW_cold/2(HX_parameters)
  [Fin_parameters] -> Thermal_resistance_KpW_cold/3(Fin_parameters)
  [HTC_Wpm2K_cold] -> Thermal_resistance_KpW_cold/1(Convective_HTC)
  [HX_parameters] -> Thermal_resistance_KpW_hot/2(HX_parameters)
  [Fin_parameters] -> Thermal_resistance_KpW_hot/3(Fin_parameters)
  [HTC_Wpm2K_hot] -> Thermal_resistance_KpW_hot/1(Convective_HTC)
  convective_HTC_Wm-2K-1_cold/1(Convective_HTC_Wm-2K-1) -> [HTC_Wpm2K_cold]
  convective_HTC_Wm-2K-1_hot/1(Convective_HTC_Wm-2K-1) -> [HTC_Wpm2K_hot]
  Pressure_drop_cold/2(pres_Pa) -> [pres_Pa_out_cold]
  Pressure_drop_hot/2(pres_Pa) -> [pres_Pa_out_hot]
  Pressure_drop_cold/1(pres_drop_Pa) -> [delta_pres_Pa_cold]
  Pressure_drop_hot/1(pres_drop_Pa) -> [delta_pres_Pa_hot]
  Colburn_J_factor_cold/1(Colburn_J_factor) -> convective_HTC_Wm-2K-1_cold/1(Colburn_J_factor), [Colburn_J_factor_cold]
  [Hydraulic_diam_m] -> convective_HTC_Wm-2K-1_cold/4(hydraulic_diameter)
  [air_properties_in_cold] -> convective_HTC_Wm-2K-1_cold/3(air_properties)
  [Re_number_in_cold] -> convective_HTC_Wm-2K-1_cold/2(Re)
  [Hydraulic_diam_m] -> convective_HTC_Wm-2K-1_hot/4(hydraulic_diameter)
  [air_properties_in_hot] -> convective_HTC_Wm-2K-1_hot/3(air_properties)
  [Re_number_in_hot] -> convective_HTC_Wm-2K-1_hot/2(Re)
  Colburn_J_factor_hot/1(Colburn_J_factor) -> convective_HTC_Wm-2K-1_hot/1(Colburn_J_factor), [Colburn_J_factor_hot]
  Friction_factor_cold/1(Friction_factor) -> Pressure_drop_cold/1(Friction_factor), [Fricn_factor_cold]
  [In_flow_bus_cold] -> Pressure_drop_cold/6(In_flow_bus)
  [Hydraulic_diam_m] -> Pressure_drop_cold/5(D_hydraulic)
  [v_in_mps_cold] -> Pressure_drop_cold/4(air_velocity)
  [air_properties_in_cold] -> Pressure_drop_cold/3(air_properties)
  [HX_parameters] -> Pressure_drop_cold/2(HX_parameters)
  [In_flow_bus_hot] -> Pressure_drop_hot/6(In_flow_bus)
  Friction_factor_hot/1(Friction_factor) -> Pressure_drop_hot/1(Friction_factor), [Fricn_factor_hot]
  [Hydraulic_diam_m] -> Pressure_drop_hot/5(D_hydraulic)
  [v_in_mps_hot] -> Pressure_drop_hot/4(air_velocity)
  [air_properties_in_hot] -> Pressure_drop_hot/3(air_properties)
  [HX_parameters] -> Pressure_drop_hot/2(HX_parameters)
  Re_number_in_hot/2(velo_air_ms-1) -> [v_in_mps_hot]
  [Re_number_in_cold] -> Colburn_J_factor_cold/2(Re)
  [Fin_parameters_ratios] -> Colburn_J_factor_cold/1(Fin_prameter_ratios)
  [Re_number_in_cold] -> Friction_factor_cold/2(Re)
  [Fin_parameters_ratios] -> Friction_factor_cold/1(Fin_prameter_ratios)
  [Re_number_in_hot] -> Colburn_J_factor_hot/2(Re)
  [Fin_parameters_ratios] -> Colburn_J_factor_hot/1(Fin_prameter_ratios)
  [Re_number_in_hot] -> Friction_factor_hot/2(Re)
  [Fin_parameters_ratios] -> Friction_factor_hot/1(Fin_prameter_ratios)
  HX_and_Fin_paramters/3(Fin_parameters_ratios) -> [Fin_parameters_ratios]
  [air_properties_in_cold] -> Re_number_in_cold/2(air_properties)
  [In_flow_bus_cold] -> Re_number_in_cold/1(In_flow_bus)
  [HX_parameters] -> Re_number_in_cold/4(HX_paramters), Re_number_in_hot/4(HX_paramters)
  [Hydraulic_diam_m] -> Re_number_in_cold/3(Hydraulic_diam), Re_number_in_hot/3(Hydraulic_diam)
  [air_properties_in_hot] -> Re_number_in_hot/2(air_properties)
  [In_flow_bus_hot] -> Re_number_in_hot/1(In_flow_bus)
  [In_flow_bus_cold] -> Air_properties_in_flows_hot_and_cold/2(In_flow_bus_cold)
  [In_flow_bus_hot] -> Air_properties_in_flows_hot_and_cold/1(In_flow_bus_hot)
  Air_properties_in_flows_hot_and_cold/2(air_properties_in_cold1) -> [air_properties_in_cold]
  Air_properties_in_flows_hot_and_cold/1(air_properties_in_hot1) -> [air_properties_in_hot]
  HX_and_Fin_paramters/2(Fin_parameters1) -> [Fin_parameters]
  HX_and_Fin_paramters/1(HX_parameters2) -> [HX_parameters]
  Re_number_in_cold/1(Re_number) -> [Re_number_in_cold]
  Re_number_in_hot/1(Re_number) -> [Re_number_in_hot]
  Hydraulic_diam_m/1(Out1) -> [Hydraulic_diam_m]
  [Fin_parameters] -> Hydraulic_diam_m/1(Fin_parameters)
  C to K/1 -> Bus Creator/1  "temp_K"
  Pa to kPa/1 -> Bus Creator/2  "pres_kPa"
  C to K1/1 -> Bus Creator1/1  "temp_K"
  Pa to kPa1/1 -> Bus Creator1/2  "pres_kPa"
  [Heat_rate_cold_Watt] -> Bus Creator2/13  "Heat_rate_cold_Watt"
  [Heat_rate_hot_Watt] -> Bus Creator2/12  "Heat_rate_hot_Watt"
  [Core_mass_temp_C] -> Bus Creator2/11  "HX_core_mass_temp_C"
  [Fricn_factor_hot] -> Bus Creator2/3  "f_hot"
  [Fricn_factor_cold] -> Bus Creator2/4  "f_cold"
  [Colburn_J_factor_hot] -> Bus Creator2/5  "J_hot"
  [Colburn_J_factor_cold] -> Bus Creator2/6  "J_cold"
  [HTC_Wpm2K_hot] -> Bus Creator2/7  "h_hot"
  [HTC_Wpm2K_cold] -> Bus Creator2/8  "h_cold"
  [delta_pres_Pa_hot] -> Bus Creator2/9  "Delta_P_hot"
  [delta_pres_Pa_cold] -> Bus Creator2/10  "Delta_P_cold"
  [Re_number_in_hot] -> Bus Creator2/1  "Re_hot"
  [Re_number_in_cold] -> Bus Creator2/2  "Re_cold"
  In_flow_bus_hot/1 -> Bus Selector4/1
  Bus Selector4/1 -> Bus Creator3/1  "<mdot_kgps>"
  Bus Selector4/2 -> K to C/1  "<temp_K>"
  Bus Selector4/3 -> kPa to Pa/1  "<pres_kPa>"
  K to C/1 -> Bus Creator3/2  "temp_C"
  Bus Creator3/1 -> [In_flow_bus_hot]
  kPa to Pa/1 -> Bus Creator3/3  "pres_Pa"
  Bus Selector5/1 -> Bus Creator4/1  "<mdot_kgps>"
  Bus Selector5/2 -> K to C1/1  "<temp_K>"
  Bus Selector5/3 -> kPa to Pa1/1  "<pres_kPa>"
  K to C1/1 -> Bus Creator4/2  "temp_C"
  kPa to Pa1/1 -> Bus Creator4/3  "press_Pa"
  Bus Creator4/1 -> [In_flow_bus_cold]
  [T_h_av_degreeC] -> Bus Creator2/14  "T_av_hot_C"
  [T_c_av_degreeC] -> Bus Creator2/15  "T_av_cold_C"
  In_flow_bus_cold/1 -> Bus Selector5/1
